simulink model "sim_tnse_2024_pos_ctrl"  (R2020a)
settings: Solver=ode4  StartTime=0.0  StopTime=30.0  FixedStep=0.01  RelTol=1e-3
values from neighbouring files (symbols this model uses):
  alfa_theta = 20    [init_tnse_2024_pos_ctrl.m]
  c1 = diag( [ 150.0, 120.0, 120.0 ] )    [init_tnse_2024_pos_ctrl.m]
  c1_diff_sigma_bar_v = diag([25; 30; 20])    [init_tnse_2024_pos_ctrl.m]
  c1v = diag([5.8; 6.5; 6.5])    [init_tnse_2024_pos_ctrl.m]
  c2 = diag( [ 80.0, 50.0, 50.0 ] )    [init_tnse_2024_pos_ctrl.m]
  c2_diff_sigma_bar_v = diag([50; 50; 10])    [init_tnse_2024_pos_ctrl.m]
  c2v = diag([5.8; 6.5; 6.5])    [init_tnse_2024_pos_ctrl.m]
  c3_diff_sigma_bar_v = diag([15; 15; 10])    [init_tnse_2024_pos_ctrl.m]
  c3v = diag([4.8; 6.4; 6.0])    [init_tnse_2024_pos_ctrl.m]
  dp_aa_t = 0.2 * ones(3, 5) + ( 1.0 - 0.2 ) * rand(3, 5)    [init_tnse_2024_pos_ctrl.m]
  dp_ff_t = [ 0.4 * ones(1, 5) + ( 1.0 - 0.4 ) * rand(1, 5);                      0.4 * ones(1, 5) + ( 1.0 - 0.4 ) * rand(1, 5);                      0.2 * ones(1, 5) + ( 0.6 - 0.2 ) * rand(1, 5) ]    [init_tnse_2024_pos_ctrl.m]
  dp_phi_t = ( - pi / 2 ) * ones(3, 5) + ( pi / 2 - ( - pi / 2 ) ) * rand(3, 5)    [init_tnse_2024_pos_ctrl.m]
  eps0 = [0.05; 0.01; 0.01]    [init_tnse_2024_pos_ctrl.m]
  etai_0 = zeros(3,5)    [init_tnse_2024_pos_ctrl.m]
  kai0 = [15; 10; 10]    [init_tnse_2024_pos_ctrl.m]
  kai_1_t = 0.02    [init_tnse_2024_pos_ctrl.m]
  kai_3_t = 0.1    [init_tnse_2024_pos_ctrl.m]
  ksii_0 = zeros(3,5)    [init_tnse_2024_pos_ctrl.m]
  lam0 = [15; 10; 10]    [init_tnse_2024_pos_ctrl.m]
  Lamd_diff_sigma_bar_v = 0.5    [init_tnse_2024_pos_ctrl.m]
  mass_i = zeros(1,NF)    [init_tnse_2024_pos_ctrl.m]
  Mii = diag([1;0;0;0;1])    [init_tnse_2024_pos_ctrl.m]
  pos0 = zeros(3, 1)    [init_tnse_2024_pos_ctrl.m]
  PZ0 = P0(3)    [init_tnse_2024_pos_ctrl.m]
  PZ1 = 10    [init_tnse_2024_pos_ctrl.m]
  Qci_init = repmat([1;0;0;0],1,NF)    [init_tnse_2024_pos_ctrl.m]
  R0 = 4    [init_tnse_2024_pos_ctrl.m]
  R1 = 8    [init_tnse_2024_pos_ctrl.m]
  Rx2 = 10    [init_tnse_2024_pos_ctrl.m]
  Ry2 = 6    [init_tnse_2024_pos_ctrl.m]
  Rz2 = 4    [init_tnse_2024_pos_ctrl.m]
  sat_sr_low = [-30, -30, -30]    [init_tnse_2024_pos_ctrl.m]
  sat_sr_up = [30, 30, 30]    [init_tnse_2024_pos_ctrl.m]
  T0 = 0    [init_tnse_2024_pos_ctrl.m]
  T1 = tseq1    (= 10)    [init_tnse_2024_pos_ctrl.m]
  T12 = tseq1 + tseq12    (= 20)    [init_tnse_2024_pos_ctrl.m]
  T2 = tseq1 + tseq12 + tseq2    (= 30)    [init_tnse_2024_pos_ctrl.m]
  theta0 = ( 2 / 5 ) * pi    (= 1.25663706144)    [init_tnse_2024_pos_ctrl.m]
  vel0 = zeros(3, 1)    [init_tnse_2024_pos_ctrl.m]
  Wij = [0,0,1,0,0;              0,0,1,1,0;              1,0,0,0,1;              0,1,1,0,0;              0,0,1,0,0]    [init_tnse_2024_pos_ctrl.m]
  X1 = 8    [init_tnse_2024_pos_ctrl.m]
  X2 = 2    [init_tnse_2024_pos_ctrl.m]
  X3 = 3    [init_tnse_2024_pos_ctrl.m]
  Y1 = 10    [init_tnse_2024_pos_ctrl.m]
  Y2 = 2    [init_tnse_2024_pos_ctrl.m]
  Y3 = 4    [init_tnse_2024_pos_ctrl.m]
  Z1 = 4    [init_tnse_2024_pos_ctrl.m]
  Z2 = -6    [init_tnse_2024_pos_ctrl.m]
  Z3 = 2    [init_tnse_2024_pos_ctrl.m]
  zeta_diff_sigma_bar_v = 0.08    [init_tnse_2024_pos_ctrl.m]
undefined symbols (not defined in the file or in its folder): cal_frac_squ, p_alfav1, p_alfav2, q_alfav1, q_alfav2
(part 3 of 4)

== matlab function sim_tnse_2024_pos_ctrl/cal differentiator d_sigma_bar_v_hat agent 4/cal sig ==
  data: x input; z output; y input
function z = fcn(x, y)
z = x(:) .* sign(y(:));

== matlab function sim_tnse_2024_pos_ctrl/Phi_sec_sigma_i agent 1 ==
  data: sigma_i_vec input; Phi_sec_sigma_1 output
function Phi_sec_sigma_1 = fcn(sigma_i_vec)
%%%% 跟随者期望速度分布式观测器
iiuav = 1;
Phi_sec_sigma_1 = diag( [ sech( sigma_i_vec(1,iiuav) ) ^ 2, ...
                                                sech( sigma_i_vec(2,iiuav) ) ^ 2, ...
                                                sech( sigma_i_vec(3,iiuav) ) ^ 2 ] );

== matlab function sim_tnse_2024_pos_ctrl/cal differentiator d_sigma_bar_v_hat agent 4/cal sig1 ==
  data: x input; z output; y input
function z = fcn(x, y)
z = x(:) .* sign(y(:));

== matlab function sim_tnse_2024_pos_ctrl/cal differentiator d_sigma_bar_v_hat agent 4/cal sig2 ==
  data: x input; z output; y input
function z = fcn(x, y)
z = x(:) .* sign(y(:));

== matlab function sim_tnse_2024_pos_ctrl/cal differentiator d_sigma_bar_v_hat agent 4/cal sig3 ==
  data: x input; z output; y input
function z = fcn(x, y)
z = x(:) .* sign(y(:));

== matlab function sim_tnse_2024_pos_ctrl/cal differentiator d_sigma_bar_v_hat agent 4/cal sig4 ==
  data: x input; z output; y input
function z = fcn(x, y)
z = x(:) .* sign(y(:));

== matlab function sim_tnse_2024_pos_ctrl/cal differentiator d_sigma_bar_v_hat agent 4/cal sig5 ==
  data: x input; z output; y input
function z = fcn(x, y)
z = x(:) .* sign(y(:));

== matlab function sim_tnse_2024_pos_ctrl/cal differentiator d_sigma_bar_v_hat agent 4/choose sigma_bar_v ==
  data: x input; y output
function y = fcn(x)
iiuav = 4;
y = x(:,iiuav);

== matlab function sim_tnse_2024_pos_ctrl/cal differentiator d_sigma_bar_v_hat agent 4/trans to column20 ==
  data: x input; y output
function y = fcn(x)
y = x(:);

== matlab function sim_tnse_2024_pos_ctrl/cal differentiator d_sigma_bar_v_hat agent 4/trans to column21 ==
  data: x input; y output
function y = fcn(x)
y = x(:);

== matlab function sim_tnse_2024_pos_ctrl/cal differentiator d_sigma_bar_v_hat agent 4/trans to column22 ==
  data: x input; y output
function y = fcn(x)
y = x(:);

== matlab function sim_tnse_2024_pos_ctrl/cal differentiator d_sigma_bar_v_hat agent 4/trans to column23 ==
  data: x input; y output
function y = fcn(x)
y = x(:);

== matlab function sim_tnse_2024_pos_ctrl/Phi_sec_sigma_i agent 2 ==
  data: sigma_i_vec input; Phi_sec_sigma_2 output
function Phi_sec_sigma_2 = fcn(sigma_i_vec)
%%%% 跟随者期望速度分布式观测器
iiuav = 2;
Phi_sec_sigma_2 = diag( [ sech( sigma_i_vec(1,iiuav) ) ^ 2, ...
                                                sech( sigma_i_vec(2,iiuav) ) ^ 2, ...
                                                sech( sigma_i_vec(3,iiuav) ) ^ 2 ] );

== matlab function sim_tnse_2024_pos_ctrl/cal Rci from ui ==
  data: Rci output; mi_vec input; ui_vec input
function Rci = fcn(mi_vec, ui_vec)
Rci = zeros(3,3,5);
for iiuav = 1:5
    Rci(:,:,iiuav) = cal_Rc_with_u(mi_vec(iiuav), ui_vec(:,iiuav));
end

end

== matlab function sim_tnse_2024_pos_ctrl/cal differentiator d_sigma_bar_v_hat agent 4/trans to column24 ==
  data: x input; y output
function y = fcn(x)
y = x(:);

== matlab function sim_tnse_2024_pos_ctrl/cal differentiator d_sigma_bar_v_hat agent 4/trans to column25 ==
  data: x input; y output
function y = fcn(x)
y = x(:);

== matlab function sim_tnse_2024_pos_ctrl/cal differentiator d_sigma_bar_v_hat agent 5/cal differentiator ==
  data: c1 input; d_sigma_bar_v_hat output; d_dsigma_bar_v_hat output; d_d2sigma_bar_v_hat output; c2 input; c3 input; chi_t input; sigma_bar_v_sig_1 input; sigma_bar_v_sig_2 input; sigma_bar_v_sig_3 input; sigma_bar_v_sig_4 input; sigma_bar_v_sig_5 input; sigma_bar_v_sig_6 input; d_sigma_bar_v_hat input; d2_sigma_bar_v_hat input
function [d_sigma_bar_v_hat, d_dsigma_bar_v_hat, d_d2sigma_bar_v_hat] = fcn(c1, c2, c3, chi_t, sigma_bar_v_sig_1, sigma_bar_v_sig_2, sigma_bar_v_sig_3, ...
                                                                                                                                                sigma_bar_v_sig_4, sigma_bar_v_sig_5, sigma_bar_v_sig_6, d_sigma_bar_v_hat, d2_sigma_bar_v_hat)
d_d2sigma_bar_v_hat = -chi_t .* c1 * sigma_bar_v_sig_1(:) - (1 - chi_t) .* c1 * sigma_bar_v_sig_2(:);
d_dsigma_bar_v_hat = -chi_t .* c2 * sigma_bar_v_sig_3(:) - (1 - chi_t) .* c2 * sigma_bar_v_sig_4(:) + d2_sigma_bar_v_hat(:);
d_sigma_bar_v_hat = -chi_t .* c3 * sigma_bar_v_sig_5(:) - (1 - chi_t) .* c3 * sigma_bar_v_sig_6(:) + d_sigma_bar_v_hat(:);

== matlab function sim_tnse_2024_pos_ctrl/cal differentiator d_sigma_bar_v_hat agent 5/cal sig ==
  data: x input; z output; y input
function z = fcn(x, y)
z = x(:) .* sign(y(:));

== matlab function sim_tnse_2024_pos_ctrl/cal differentiator d_sigma_bar_v_hat agent 5/cal sig1 ==
  data: x input; z output; y input
function z = fcn(x, y)
z = x(:) .* sign(y(:));

== matlab function sim_tnse_2024_pos_ctrl/cal differentiator d_sigma_bar_v_hat agent 5/cal sig2 ==
  data: x input; z output; y input
function z = fcn(x, y)
z = x(:) .* sign(y(:));

== matlab function sim_tnse_2024_pos_ctrl/Phi_sec_sigma_i agent 3 ==
  data: sigma_i_vec input; Phi_sec_sigma_3 output
function Phi_sec_sigma_3 = fcn(sigma_i_vec)
%%%% 跟随者期望速度分布式观测器
iiuav = 3;
Phi_sec_sigma_3 = diag( [ sech( sigma_i_vec(1,iiuav) ) ^ 2, ...
                                                sech( sigma_i_vec(2,iiuav) ) ^ 2, ...
                                                sech( sigma_i_vec(3,iiuav) ) ^ 2 ] );

== matlab function sim_tnse_2024_pos_ctrl/cal differentiator d_sigma_bar_v_hat agent 5/cal sig3 ==
  data: x input; z output; y input
function z = fcn(x, y)
z = x(:) .* sign(y(:));

== matlab function sim_tnse_2024_pos_ctrl/cal differentiator d_sigma_bar_v_hat agent 5/cal sig4 ==
  data: x input; z output; y input
function z = fcn(x, y)
z = x(:) .* sign(y(:));

== matlab function sim_tnse_2024_pos_ctrl/cal differentiator d_sigma_bar_v_hat agent 5/cal sig5 ==
  data: x input; z output; y input
function z = fcn(x, y)
z = x(:) .* sign(y(:));

== matlab function sim_tnse_2024_pos_ctrl/cal differentiator d_sigma_bar_v_hat agent 5/choose sigma_bar_v ==
  data: x input; y output
function y = fcn(x)
iiuav = 5;
y = x(:,iiuav);

== matlab function sim_tnse_2024_pos_ctrl/cal differentiator d_sigma_bar_v_hat agent 5/trans to column20 ==
  data: x input; y output
function y = fcn(x)
y = x(:);

== matlab function sim_tnse_2024_pos_ctrl/cal differentiator d_sigma_bar_v_hat agent 5/trans to column21 ==
  data: x input; y output
function y = fcn(x)
y = x(:);

== matlab function sim_tnse_2024_pos_ctrl/cal differentiator d_sigma_bar_v_hat agent 5/trans to column22 ==
  data: x input; y output
function y = fcn(x)
y = x(:);

== matlab function sim_tnse_2024_pos_ctrl/cal differentiator d_sigma_bar_v_hat agent 5/trans to column23 ==
  data: x input; y output
function y = fcn(x)
y = x(:);

== matlab function sim_tnse_2024_pos_ctrl/cal differentiator d_sigma_bar_v_hat agent 5/trans to column24 ==
  data: x input; y output
function y = fcn(x)
y = x(:);

== matlab function sim_tnse_2024_pos_ctrl/cal differentiator d_sigma_bar_v_hat agent 5/trans to column25 ==
  data: x input; y output
function y = fcn(x)
y = x(:);

== matlab function sim_tnse_2024_pos_ctrl/Phi_sec_sigma_i agent 4 ==
  data: sigma_i_vec input; Phi_sec_sigma_4 output
function Phi_sec_sigma_4 = fcn(sigma_i_vec)
%%%% 跟随者期望速度分布式观测器
iiuav = 4;
Phi_sec_sigma_4 = diag( [ sech( sigma_i_vec(1,iiuav) ) ^ 2, ...
                                                sech( sigma_i_vec(2,iiuav) ) ^ 2, ...
                                                sech( sigma_i_vec(3,iiuav) ) ^ 2 ] );

== matlab function sim_tnse_2024_pos_ctrl/combine d_sigma_bar_v_est ==
  data: d_sigma_bar_v_est_1 input; d_sigma_bar_v_est_2 input; d_sigma_bar_v_est_3 input; d_sigma_bar_v_est_4 input; d_sigma_bar_v_est_5 input; d_sigma_bar_v_vec output
function d_sigma_bar_v_vec  = fcn(d_sigma_bar_v_est_1, d_sigma_bar_v_est_2, d_sigma_bar_v_est_3, d_sigma_bar_v_est_4, d_sigma_bar_v_est_5)
%%%% 合并用微分器求得的虚拟速度控制量导数
d_sigma_bar_v_vec = [d_sigma_bar_v_est_1(:), d_sigma_bar_v_est_2(:), d_sigma_bar_v_est_3(:), d_sigma_bar_v_est_4(:), d_sigma_bar_v_est_5(:)];

== matlab function sim_tnse_2024_pos_ctrl/cal abs 21 ==
  data: x input; y output
function y = fcn(x)
y = abs(x(:));

== matlab function sim_tnse_2024_pos_ctrl/cal abs 22 ==
  data: x input; y output
function y = fcn(x)
y = abs(x(:));

== matlab function sim_tnse_2024_pos_ctrl/choose ksi_est_err 21 ==
  data: x input; y output
function y = fcn(x)
iiuav = 1;
y = x(:,iiuav);

== matlab function sim_tnse_2024_pos_ctrl/choose ksi_est_err 22 ==
  data: x input; y output
function y = fcn(x)
iiuav = 1;
y = x(:,iiuav);

== matlab function sim_tnse_2024_pos_ctrl/trans to column20 ==
  data: x input; y output
function y = fcn(x)
y = x(:);

== matlab function sim_tnse_2024_pos_ctrl/trans to column21 ==
  data: x input; y output
function y = fcn(x)
y = x(:);

== matlab function sim_tnse_2024_pos_ctrl/cal theta_sigma_bar_v_tilt agent 1 ==
  data: alfa_theta input; sigma_bar_v_tilt_squ_1_1 input; theta_sigma_bar_v_tilt_1_1 output; sigma_bar_v_tilt_squ_2_1 input; sigma_bar_v_tilt_vec input; theta_sigma_bar_v_tilt_2_1 output
function [theta_sigma_bar_v_tilt_1_1, theta_sigma_bar_v_tilt_2_1] = fcn(alfa_theta, sigma_bar_v_tilt_squ_1_1, sigma_bar_v_tilt_squ_2_1, sigma_bar_v_tilt_vec)
%%%% 计算平滑递增函数
iiuav = 1;
theta_sigma_bar_v_tilt_1_1 = sigma_bar_v_tilt_squ_1_1(:) .* ( -1 + 2 ./ ( 1 + exp( -alfa_theta .* sigma_bar_v_tilt_vec(:,iiuav) ) ) );
theta_sigma_bar_v_tilt_2_1 = sigma_bar_v_tilt_squ_2_1(:) .* ( -1 + 2 ./ ( 1 + exp( -alfa_theta .* sigma_bar_v_tilt_vec(:,iiuav) ) ) );

== matlab function sim_tnse_2024_pos_ctrl/cal abs 23 ==
  data: x input; y output
function y = fcn(x)
y = abs(x(:));

== matlab function sim_tnse_2024_pos_ctrl/Phi_sec_sigma_i agent 5 ==
  data: sigma_i_vec input; Phi_sec_sigma_5 output
function Phi_sec_sigma_5 = fcn(sigma_i_vec)
%%%% 跟随者期望速度分布式观测器
iiuav = 5;
Phi_sec_sigma_5 = diag( [ sech( sigma_i_vec(1,iiuav) ) ^ 2, ...
                                                sech( sigma_i_vec(2,iiuav) ) ^ 2, ...
                                                sech( sigma_i_vec(3,iiuav) ) ^ 2 ] );

== matlab function sim_tnse_2024_pos_ctrl/cal abs 24 ==
  data: x input; y output
function y = fcn(x)
y = abs(x(:));

== matlab function sim_tnse_2024_pos_ctrl/cal theta_sigma_bar_v_tilt agent 2 ==
  data: alfa_theta input; sigma_bar_v_tilt_squ_1_2 input; theta_sigma_bar_v_tilt_1_2 output; sigma_bar_v_tilt_squ_2_2 input; sigma_bar_v_tilt_vec input; theta_sigma_bar_v_tilt_2_2 output
function [theta_sigma_bar_v_tilt_1_2, theta_sigma_bar_v_tilt_2_2] = fcn(alfa_theta, sigma_bar_v_tilt_squ_1_2, sigma_bar_v_tilt_squ_2_2, sigma_bar_v_tilt_vec)
%%%% 计算平滑递增函数
iiuav = 2;
theta_sigma_bar_v_tilt_1_2 = sigma_bar_v_tilt_squ_1_2(:) .* ( -1 + 2 ./ ( 1 + exp( -alfa_theta .* sigma_bar_v_tilt_vec(:,iiuav) ) ) );
theta_sigma_bar_v_tilt_2_2 = sigma_bar_v_tilt_squ_2_2(:) .* ( -1 + 2 ./ ( 1 + exp( -alfa_theta .* sigma_bar_v_tilt_vec(:,iiuav) ) ) );

== matlab function sim_tnse_2024_pos_ctrl/choose ksi_est_err 23 ==
  data: x input; y output
function y = fcn(x)
iiuav = 2;
y = x(:,iiuav);

== matlab function sim_tnse_2024_pos_ctrl/choose ksi_est_err 24 ==
  data: x input; y output
function y = fcn(x)
iiuav = 2;
y = x(:,iiuav);

== matlab function sim_tnse_2024_pos_ctrl/trans to column22 ==
  data: x input; y output
function y = fcn(x)
y = x(:);

== matlab function sim_tnse_2024_pos_ctrl/trans to column23 ==
  data: x input; y output
function y = fcn(x)
y = x(:);

== matlab function sim_tnse_2024_pos_ctrl/cal abs 25 ==
  data: x input; y output
function y = fcn(x)
y = abs(x(:));

== matlab function sim_tnse_2024_pos_ctrl/cal abs 26 ==
  data: x input; y output
function y = fcn(x)
y = abs(x(:));

== matlab function sim_tnse_2024_pos_ctrl/cal theta_sigma_bar_v_tilt agent 3 ==
  data: alfa_theta input; sigma_bar_v_tilt_squ_1_3 input; theta_sigma_bar_v_tilt_1_3 output; sigma_bar_v_tilt_squ_2_3 input; sigma_bar_v_tilt_vec input; theta_sigma_bar_v_tilt_2_3 output
function [theta_sigma_bar_v_tilt_1_3, theta_sigma_bar_v_tilt_2_3] = fcn(alfa_theta, sigma_bar_v_tilt_squ_1_3, sigma_bar_v_tilt_squ_2_3, sigma_bar_v_tilt_vec)
%%%% 计算平滑递增函数
iiuav = 3;
theta_sigma_bar_v_tilt_1_3 = sigma_bar_v_tilt_squ_1_3(:) .* ( -1 + 2 ./ ( 1 + exp( -alfa_theta .* sigma_bar_v_tilt_vec(:,iiuav) ) ) );
theta_sigma_bar_v_tilt_2_3 = sigma_bar_v_tilt_squ_2_3(:) .* ( -1 + 2 ./ ( 1 + exp( -alfa_theta .* sigma_bar_v_tilt_vec(:,iiuav) ) ) );

== matlab function sim_tnse_2024_pos_ctrl/combine betai ==
  data: beta_hat_1 input; beta_hat_vec output; beta_hat_2 input; beta_hat_3 input; beta_hat_4 input; beta_hat_5 input
function beta_hat_vec  = fcn(beta_hat_1, beta_hat_2, beta_hat_3, beta_hat_4, beta_hat_5)
%%%% 合并自适应律
beta_hat_vec = [beta_hat_1, beta_hat_2, beta_hat_3, beta_hat_4, beta_hat_5];

== matlab function sim_tnse_2024_pos_ctrl/choose ksi_est_err 25 ==
  data: x input; y output
function y = fcn(x)
iiuav = 3;
y = x(:,iiuav);

== matlab function sim_tnse_2024_pos_ctrl/choose ksi_est_err 26 ==
  data: x input; y output
function y = fcn(x)
iiuav = 3;
y = x(:,iiuav);

== matlab function sim_tnse_2024_pos_ctrl/trans to column24 ==
  data: x input; y output
function y = fcn(x)
y = x(:);

== matlab function sim_tnse_2024_pos_ctrl/trans to column25 ==
  data: x input; y output
function y = fcn(x)
y = x(:);

== matlab function sim_tnse_2024_pos_ctrl/cal abs 27 ==
  data: x input; y output
function y = fcn(x)
y = abs(x(:));

== matlab function sim_tnse_2024_pos_ctrl/cal abs 28 ==
  data: x input; y output
function y = fcn(x)
y = abs(x(:));

== matlab function sim_tnse_2024_pos_ctrl/cal theta_sigma_bar_v_tilt agent 4 ==
  data: alfa_theta input; sigma_bar_v_tilt_squ_1_4 input; theta_sigma_bar_v_tilt_1_4 output; sigma_bar_v_tilt_squ_2_4 input; sigma_bar_v_tilt_vec input; theta_sigma_bar_v_tilt_2_4 output
function [theta_sigma_bar_v_tilt_1_4, theta_sigma_bar_v_tilt_2_4] = fcn(alfa_theta, sigma_bar_v_tilt_squ_1_4, sigma_bar_v_tilt_squ_2_4, sigma_bar_v_tilt_vec)
%%%% 计算平滑递增函数
iiuav = 4;
theta_sigma_bar_v_tilt_1_4 = sigma_bar_v_tilt_squ_1_4(:) .* ( -1 + 2 ./ ( 1 + exp( -alfa_theta .* sigma_bar_v_tilt_vec(:,iiuav) ) ) );
theta_sigma_bar_v_tilt_2_4 = sigma_bar_v_tilt_squ_2_4(:) .* ( -1 + 2 ./ ( 1 + exp( -alfa_theta .* sigma_bar_v_tilt_vec(:,iiuav) ) ) );

== matlab function sim_tnse_2024_pos_ctrl/choose ksi_est_err 27 ==
  data: x input; y output
function y = fcn(x)
iiuav = 4;
y = x(:,iiuav);

== matlab function sim_tnse_2024_pos_ctrl/choose ksi_est_err 28 ==
  data: x input; y output
function y = fcn(x)
iiuav = 4;
y = x(:,iiuav);

== matlab function sim_tnse_2024_pos_ctrl/trans to column26 ==
  data: x input; y output
function y = fcn(x)
y = x(:);

== matlab function sim_tnse_2024_pos_ctrl/trans to column27 ==
  data: x input; y output
function y = fcn(x)
y = x(:);

== matlab function sim_tnse_2024_pos_ctrl/cal abs 29 ==
  data: x input; y output
function y = fcn(x)
y = abs(x(:));

== matlab function sim_tnse_2024_pos_ctrl/cal abs 30 ==
  data: x input; y output
function y = fcn(x)
y = abs(x(:));

== matlab function sim_tnse_2024_pos_ctrl/cal theta_sigma_bar_v_tilt agent 5 ==
  data: alfa_theta input; sigma_bar_v_tilt_squ_1_5 input; theta_sigma_bar_v_tilt_1_5 output; sigma_bar_v_tilt_squ_2_5 input; sigma_bar_v_tilt_vec input; theta_sigma_bar_v_tilt_2_5 output
function [theta_sigma_bar_v_tilt_1_5, theta_sigma_bar_v_tilt_2_5] = fcn(alfa_theta, sigma_bar_v_tilt_squ_1_5, sigma_bar_v_tilt_squ_2_5, sigma_bar_v_tilt_vec)
%%%% 计算平滑递增函数
iiuav = 5;
theta_sigma_bar_v_tilt_1_5 = sigma_bar_v_tilt_squ_1_5(:) .* ( -1 + 2 ./ ( 1 + exp( -alfa_theta .* sigma_bar_v_tilt_vec(:,iiuav) ) ) );
theta_sigma_bar_v_tilt_2_5 = sigma_bar_v_tilt_squ_2_5(:) .* ( -1 + 2 ./ ( 1 + exp( -alfa_theta .* sigma_bar_v_tilt_vec(:,iiuav) ) ) );

== matlab function sim_tnse_2024_pos_ctrl/update betai agent 1 ==
  data: eps0 input; d_beta_hat_1 output; Wij input; Mii input; tsim input; u0 input; rho_hat_vec input
function d_beta_hat_1 = fcn(eps0, Wij, Mii, tsim, u0, rho_hat_vec)
%%%% 自适应律
iiuav = 1;
err_rho = Mii(iiuav, iiuav) * ( rho_hat_vec(:,iiuav) - u0(:) );
for jjuav = 1:5
    err_rho = err_rho + Wij(iiuav, jjuav) * ( rho_hat_vec(:,iiuav) - rho_hat_vec(:,jjuav) );
end
d_beta_hat_1 = ( err_rho(:)' ) * tanh( err_rho(:) ./ exp( -eps0 * tsim ) );

== matlab function sim_tnse_2024_pos_ctrl/choose ksi_est_err 29 ==
  data: x input; y output
function y = fcn(x)
iiuav = 5;
y = x(:,iiuav);

== matlab function sim_tnse_2024_pos_ctrl/choose ksi_est_err 30 ==
  data: x input; y output
function y = fcn(x)
iiuav = 5;
y = x(:,iiuav);

== matlab function sim_tnse_2024_pos_ctrl/trans to column28 ==
  data: x input; y output
function y = fcn(x)
y = x(:);

== matlab function sim_tnse_2024_pos_ctrl/trans to column29 ==
  data: x input; y output
function y = fcn(x)
y = x(:);

== matlab function sim_tnse_2024_pos_ctrl/combine theta_sigma_bar_v_tilt ==
  data: theta_sigma_bar_v_tilt_1_1 input; theta_sigma_bar_v_tilt_1_2 input; theta_sigma_bar_v_tilt_1_3 input; theta_sigma_bar_v_tilt_1_4 input; theta_sigma_bar_v_tilt_1_5 input; theta_sigma_bar_v_tilt_1_vec output; theta_sigma_bar_v_tilt_2_1 input; theta_sigma_bar_v_tilt_2_vec output; theta_sigma_bar_v_tilt_2_2 input; theta_sigma_bar_v_tilt_2_3 input; theta_sigma_bar_v_tilt_2_4 input; theta_sigma_bar_v_tilt_2_5 input
function [theta_sigma_bar_v_tilt_1_vec, theta_sigma_bar_v_tilt_2_vec]  = fcn(theta_sigma_bar_v_tilt_1_1, theta_sigma_bar_v_tilt_1_2, theta_sigma_bar_v_tilt_1_3, theta_sigma_bar_v_tilt_1_4, theta_sigma_bar_v_tilt_1_5, ...
                                                                                                                                            theta_sigma_bar_v_tilt_2_1, theta_sigma_bar_v_tilt_2_2, theta_sigma_bar_v_tilt_2_3, theta_sigma_bar_v_tilt_2_4, theta_sigma_bar_v_tilt_2_5)
%%%% 合并领导者位置观测器输出结果
theta_sigma_bar_v_tilt_1_vec = [theta_sigma_bar_v_tilt_1_1(:), theta_sigma_bar_v_tilt_1_2(:), theta_sigma_bar_v_tilt_1_3(:), theta_sigma_bar_v_tilt_1_4(:), theta_sigma_bar_v_tilt_1_5(:)];
theta_sigma_bar_v_tilt_2_vec = [theta_sigma_bar_v_tilt_2_1(:), theta_sigma_bar_v_tilt_2_2(:), theta_sigma_bar_v_tilt_2_3(:), theta_sigma_bar_v_tilt_2_4(:), theta_sigma_bar_v_tilt_2_5(:)];

== matlab function sim_tnse_2024_pos_ctrl/cal sigma_bar_v_hat agent 1 ==
  data: c1v input; c2v input; theta_sigma_bar_v_tilt_1_vec input; d_sigma_bar_v_hat_1 output; theta_sigma_bar_v_tilt_2_vec input; d_sigma_bar_v_vec input
function d_sigma_bar_v_hat_1 = fcn(c1v, c2v, theta_sigma_bar_v_tilt_1_vec, theta_sigma_bar_v_tilt_2_vec, d_sigma_bar_v_vec)
%%%% 计算扰动观测器中虚拟速度控制量观测值sigma_v_hat的微分方程
iiuav = 1;
d_sigma_bar_v_hat_1 = d_sigma_bar_v_vec(:,iiuav) + ...
                                            c1v * theta_sigma_bar_v_tilt_1_vec(:,iiuav) + ...
                                            c2v * theta_sigma_bar_v_tilt_2_vec(:,iiuav);

== matlab function sim_tnse_2024_pos_ctrl/cal sigma_bar_v_hat agent 2 ==
  data: c1v input; c2v input; theta_sigma_bar_v_tilt_1_vec input; d_sigma_bar_v_hat_2 output; theta_sigma_bar_v_tilt_2_vec input; d_sigma_bar_v_vec input
function d_sigma_bar_v_hat_2 = fcn(c1v, c2v, theta_sigma_bar_v_tilt_1_vec, theta_sigma_bar_v_tilt_2_vec, d_sigma_bar_v_vec)
%%%% 计算扰动观测器中虚拟速度控制量观测值sigma_v_hat的微分方程
iiuav = 2;
d_sigma_bar_v_hat_2 = d_sigma_bar_v_vec(:,iiuav) + ...
                                            c1v * theta_sigma_bar_v_tilt_1_vec(:,iiuav) + ...
                                            c2v * theta_sigma_bar_v_tilt_2_vec(:,iiuav);

== matlab function sim_tnse_2024_pos_ctrl/cal sigma_bar_v_hat agent 3 ==
  data: c1v input; c2v input; theta_sigma_bar_v_tilt_1_vec input; d_sigma_bar_v_hat_3 output; theta_sigma_bar_v_tilt_2_vec input; d_sigma_bar_v_vec input
function d_sigma_bar_v_hat_3 = fcn(c1v, c2v, theta_sigma_bar_v_tilt_1_vec, theta_sigma_bar_v_tilt_2_vec, d_sigma_bar_v_vec)
%%%% 计算扰动观测器中虚拟速度控制量观测值sigma_v_hat的微分方程
iiuav = 3;
d_sigma_bar_v_hat_3 = d_sigma_bar_v_vec(:,iiuav) + ...
                                            c1v * theta_sigma_bar_v_tilt_1_vec(:,iiuav) + ...
                                            c2v * theta_sigma_bar_v_tilt_2_vec(:,iiuav);

== matlab function sim_tnse_2024_pos_ctrl/cal sigma_bar_v_hat agent 4 ==
  data: c1v input; c2v input; theta_sigma_bar_v_tilt_1_vec input; d_sigma_bar_v_hat_4 output; theta_sigma_bar_v_tilt_2_vec input; d_sigma_bar_v_vec input
function d_sigma_bar_v_hat_4 = fcn(c1v, c2v, theta_sigma_bar_v_tilt_1_vec, theta_sigma_bar_v_tilt_2_vec, d_sigma_bar_v_vec)
%%%% 计算扰动观测器中虚拟速度控制量观测值sigma_v_hat的微分方程
iiuav = 4;
d_sigma_bar_v_hat_4 = d_sigma_bar_v_vec(:,iiuav) + ...
                                            c1v * theta_sigma_bar_v_tilt_1_vec(:,iiuav) + ...
                                            c2v * theta_sigma_bar_v_tilt_2_vec(:,iiuav);

== matlab function sim_tnse_2024_pos_ctrl/cal sigma_bar_v_hat agent 5 ==
  data: c1v input; c2v input; theta_sigma_bar_v_tilt_1_vec input; d_sigma_bar_v_hat_5 output; theta_sigma_bar_v_tilt_2_vec input; d_sigma_bar_v_vec input
function d_sigma_bar_v_hat_5 = fcn(c1v, c2v, theta_sigma_bar_v_tilt_1_vec, theta_sigma_bar_v_tilt_2_vec, d_sigma_bar_v_vec)
%%%% 计算扰动观测器中虚拟速度控制量观测值sigma_v_hat的微分方程
iiuav = 5;
d_sigma_bar_v_hat_5 = d_sigma_bar_v_vec(:,iiuav) + ...
                                            c1v * theta_sigma_bar_v_tilt_1_vec(:,iiuav) + ...
                                            c2v * theta_sigma_bar_v_tilt_2_vec(:,iiuav);

== matlab function sim_tnse_2024_pos_ctrl/cal combine sigma_bar_v_tilt ==
  data: sigma_bar_v_vec input; sigma_bar_v_hat_vec input; sigma_bar_v_tilt_vec output
function sigma_bar_v_tilt_vec = fcn(sigma_bar_v_vec, sigma_bar_v_hat_vec)
%%%% 计算虚拟速度观测误差sigma_bar_v_tilt
sigma_bar_v_tilt_vec = zeros(3,5);
for iiuav = 1:5
    sigma_bar_v_tilt_vec(:,iiuav) = sigma_bar_v_vec(:,iiuav) - sigma_bar_v_hat_vec(:,iiuav);
end

== matlab function sim_tnse_2024_pos_ctrl/combine sigma_bar_v_hat ==
  data: sigma_bar_v_hat_1 input; sigma_bar_v_hat_2 input; sigma_bar_v_hat_3 input; sigma_bar_v_hat_4 input; sigma_bar_v_hat_5 input; sigma_bar_v_hat_vec output
function sigma_bar_v_hat_vec  = fcn(sigma_bar_v_hat_1, sigma_bar_v_hat_2, sigma_bar_v_hat_3, sigma_bar_v_hat_4, sigma_bar_v_hat_5)
%%%% 合并虚拟速度控制量观测值sigma_bar_v_hat
sigma_bar_v_hat_vec = [sigma_bar_v_hat_1(:), sigma_bar_v_hat_2(:), sigma_bar_v_hat_3(:), sigma_bar_v_hat_4(:), sigma_bar_v_hat_5(:)];

== matlab function sim_tnse_2024_pos_ctrl/update betai agent 2 ==
  data: eps0 input; d_beta_hat_2 output; Wij input; Mii input; tsim input; u0 input; rho_hat_vec input
function d_beta_hat_2 = fcn(eps0, Wij, Mii, tsim, u0, rho_hat_vec)
%%%% 自适应律
iiuav = 2;
err_rho = Mii(iiuav, iiuav) * ( rho_hat_vec(:,iiuav) - u0(:) );
for jjuav = 1:5
    err_rho = err_rho + Wij(iiuav, jjuav) * ( rho_hat_vec(:,iiuav) - rho_hat_vec(:,jjuav) );
end
d_beta_hat_2 = ( err_rho(:)' ) * tanh( err_rho(:) ./ exp( -eps0 * tsim ) );

== matlab function sim_tnse_2024_pos_ctrl/cal dp_hat agent 1 ==
  data: c3v input; d_sigma_bar_v_vec input; sigma_bar_v_hat_vec input; dp_hat_1 output
function dp_hat_1 = fcn(c3v, d_sigma_bar_v_vec, sigma_bar_v_hat_vec)
%%%% 计算扰动观测值dp_hat
iiuav = 1;
dp_hat_1 = d_sigma_bar_v_vec(:,iiuav) + c3v * sigma_bar_v_hat_vec(:,iiuav);

== matlab function sim_tnse_2024_pos_ctrl/cal dp_hat agent 2 ==
  data: c3v input; d_sigma_bar_v_vec input; sigma_bar_v_hat_vec input; dp_hat_2 output
function dp_hat_2 = fcn(c3v, d_sigma_bar_v_vec, sigma_bar_v_hat_vec)
%%%% 计算扰动观测值dp_hat
iiuav = 2;
dp_hat_2 = d_sigma_bar_v_vec(:,iiuav) + c3v * sigma_bar_v_hat_vec(:,iiuav);

== matlab function sim_tnse_2024_pos_ctrl/cal dp_hat agent 3 ==
  data: c3v input; d_sigma_bar_v_vec input; sigma_bar_v_hat_vec input; dp_hat_3 output
function dp_hat_3 = fcn(c3v, d_sigma_bar_v_vec, sigma_bar_v_hat_vec)
%%%% 计算扰动观测值dp_hat
iiuav = 3;
dp_hat_3 = d_sigma_bar_v_vec(:,iiuav) + c3v * sigma_bar_v_hat_vec(:,iiuav);

== matlab function sim_tnse_2024_pos_ctrl/cal dp_hat agent 4 ==
  data: c3v input; d_sigma_bar_v_vec input; sigma_bar_v_hat_vec input; dp_hat_4 output
function dp_hat_4 = fcn(c3v, d_sigma_bar_v_vec, sigma_bar_v_hat_vec)
%%%% 计算扰动观测值dp_hat
iiuav = 4;
dp_hat_4 = d_sigma_bar_v_vec(:,iiuav) + c3v * sigma_bar_v_hat_vec(:,iiuav);

== matlab function sim_tnse_2024_pos_ctrl/cal dp_hat agent 5 ==
  data: c3v input; d_sigma_bar_v_vec input; sigma_bar_v_hat_vec input; dp_hat_5 output
function dp_hat_5 = fcn(c3v, d_sigma_bar_v_vec, sigma_bar_v_hat_vec)
%%%% 计算扰动观测值dp_hat
iiuav = 5;
dp_hat_5 = d_sigma_bar_v_vec(:,iiuav) + c3v * sigma_bar_v_hat_vec(:,iiuav);

== matlab function sim_tnse_2024_pos_ctrl/combine dp_hat ==
  data: dp_hat_1 input; dp_hat_2 input; dp_hat_3 input; dp_hat_4 input; dp_hat_5 input; dp_hat_vec output
function dp_hat_vec  = fcn(dp_hat_1, dp_hat_2, dp_hat_3, dp_hat_4, dp_hat_5)
%%%% 合并扰动观测值dp_hat
dp_hat_vec = [dp_hat_1(:), dp_hat_2(:), dp_hat_3(:), dp_hat_4(:), dp_hat_5(:)];

== matlab function sim_tnse_2024_pos_ctrl/cal ui agent 1 ==
  data: c1 input; c2 input; sat_sr_up input; sat_sr_low input; ui_1 output; rho_hat_vec input; dp_hat_vec input; si_vec input; ri_vec input
function ui_1 = fcn(c1, c2, sat_sr_up, sat_sr_low, rho_hat_vec, dp_hat_vec, si_vec, ri_vec)
%%%% 计算控制输入ui
iiuav = 1;
g0 = 9.80663;
e3 = [0;0;1];
sat_si_ri = zeros(3,1);
sat_ri = zeros(3,1);
c_mul_si_ri = c1 * ( si_vec(:,iiuav) + ri_vec(:,iiuav) );
c_mul_ri = c2 * ri_vec(:,iiuav);
for jj = 1:3
    if c_mul_si_ri(jj) < sat_sr_low(jj)
        sat_si_ri(jj) = sat_sr_low(jj);
    elseif c_mul_si_ri(jj) > sat_sr_up(jj)
        sat_si_ri(jj) = sat_sr_up(jj);
    else
        sat_si_ri(jj) = c_mul_ri(jj);
    end
    if c_mul_ri(jj) < sat_sr_low(jj)
        sat_ri(jj) = sat_sr_low(jj);
    elseif c_mul_ri(jj) > sat_sr_up(jj)
        sat_ri(jj) = sat_sr_up(jj);
    else
        sat_ri(jj) = c_mul_ri(jj);
    end
end
ui_1 = g0 * e3 + rho_hat_vec(:,iiuav) - dp_hat_vec(:,iiuav) ...
            - sat_si_ri(:) - sat_ri(:);

== matlab function sim_tnse_2024_pos_ctrl/combine ui ==
  data: ui_1 input; ui_2 input; ui_3 input; ui_4 input; ui_5 input; ui_vec output
function ui_vec  = fcn(ui_1, ui_2, ui_3, ui_4, ui_5)
%%%% 合并控制输入ui
ui_vec = [ui_1(:), ui_2(:), ui_3(:), ui_4(:), ui_5(:)];

== matlab function sim_tnse_2024_pos_ctrl/cal disturbance observation error dp_tilt ==
  data: dp_vec input; dp_tilt_vec output; dp_hat_vec input
function dp_tilt_vec = fcn(dp_vec, dp_hat_vec)
%%%% 计算扰动观测器估计误差dp_tilt
dp_tilt_vec = zeros(3,5);
for iiuav = 1:5
    dp_tilt_vec(:,iiuav) = dp_vec(:,iiuav) - dp_hat_vec(:,iiuav);
end

== matlab function sim_tnse_2024_pos_ctrl/combine Phi_sec_sigma_i ==
  data: Phi_sec_sigma_1 input; Phi_sec_sigma_vec output; Phi_sec_sigma_2 input; Phi_sec_sigma_3 input; Phi_sec_sigma_4 input; Phi_sec_sigma_5 input
function Phi_sec_sigma_vec  = fcn(Phi_sec_sigma_1, Phi_sec_sigma_2, Phi_sec_sigma_3, Phi_sec_sigma_4, Phi_sec_sigma_5)
%%%% 合并领导者位置观测器输出结果
Phi_sec_sigma_vec = zeros(3,3,5);
Phi_sec_sigma_vec(:,:,1) = Phi_sec_sigma_1;
Phi_sec_sigma_vec(:,:,2) = Phi_sec_sigma_2;
Phi_sec_sigma_vec(:,:,3) = Phi_sec_sigma_3;
Phi_sec_sigma_vec(:,:,4) = Phi_sec_sigma_4;
Phi_sec_sigma_vec(:,:,5) = Phi_sec_sigma_5;

== matlab function sim_tnse_2024_pos_ctrl/update betai agent 3 ==
  data: eps0 input; d_beta_hat_3 output; Wij input; Mii input; tsim input; u0 input; rho_hat_vec input
function d_beta_hat_3 = fcn(eps0, Wij, Mii, tsim, u0, rho_hat_vec)
%%%% 自适应律
iiuav = 3;
err_rho = Mii(iiuav, iiuav) * ( rho_hat_vec(:,iiuav) - u0(:) );
for jjuav = 1:5
    err_rho = err_rho + Wij(iiuav, jjuav) * ( rho_hat_vec(:,iiuav) - rho_hat_vec(:,jjuav) );
end
d_beta_hat_3 = ( err_rho(:)' ) * tanh( err_rho(:) ./ exp( -eps0 * tsim ) );

== matlab function sim_tnse_2024_pos_ctrl/update betai agent 4 ==
  data: eps0 input; d_beta_hat_4 output; Wij input; Mii input; tsim input; u0 input; rho_hat_vec input
function d_beta_hat_4 = fcn(eps0, Wij, Mii, tsim, u0, rho_hat_vec)
%%%% 自适应律
iiuav = 4;
err_rho = Mii(iiuav, iiuav) * ( rho_hat_vec(:,iiuav) - u0(:) );
for jjuav = 1:5
    err_rho = err_rho + Wij(iiuav, jjuav) * ( rho_hat_vec(:,iiuav) - rho_hat_vec(:,jjuav) );
end
d_beta_hat_4 = ( err_rho(:)' ) * tanh( err_rho(:) ./ exp( -eps0 * tsim ) );

== matlab function sim_tnse_2024_pos_ctrl/update betai agent 5 ==
  data: eps0 input; d_beta_hat_5 output; Wij input; Mii input; tsim input; u0 input; rho_hat_vec input
function d_beta_hat_5 = fcn(eps0, Wij, Mii, tsim, u0, rho_hat_vec)
%%%% 自适应律
iiuav = 5;
err_rho = Mii(iiuav, iiuav) * ( rho_hat_vec(:,iiuav) - u0(:) );
for jjuav = 1:5
    err_rho = err_rho + Wij(iiuav, jjuav) * ( rho_hat_vec(:,iiuav) - rho_hat_vec(:,jjuav) );
end
d_beta_hat_5 = ( err_rho(:)' ) * tanh( err_rho(:) ./ exp( -eps0 * tsim ) );

== matlab function sim_tnse_2024_pos_ctrl/combine betai1 ==
  data: sigmai_1 input; sigmai_vec output; sigmai_2 input; sigmai_3 input; sigmai_4 input; sigmai_5 input
function sigmai_vec  = fcn(sigmai_1, sigmai_2, sigmai_3, sigmai_4, sigmai_5)
%%%% 合并分布式观测器变量
sigmai_vec = zeros(3,5);
sigmai_vec(:,1) = sigmai_1(:);
sigmai_vec(:,2) = sigmai_2(:);
sigmai_vec(:,3) = sigmai_3(:);
sigmai_vec(:,4) = sigmai_4(:);
sigmai_vec(:,5) = sigmai_5(:);

== matlab function sim_tnse_2024_pos_ctrl/update sigmai agent 1 ==
  data: kai0 input; lam0 input; eps0 input; d_sigmai_1 output; Wij input; Mii input; tsim input; u0 input; beta_hat_vec input; rho_hat_vec input; Phi_sec_sigma_vec input
function d_sigmai_1 = fcn(kai0, lam0, eps0, Wij, Mii, tsim, u0, beta_hat_vec, rho_hat_vec, Phi_sec_sigma_vec)
%%%% 求解分布式观测器变量
iiuav = 1;
err_rho = Mii(iiuav, iiuav) * ( rho_hat_vec(:,iiuav) - u0(:) );
for jjuav = 1:5
    err_rho = err_rho + Wij(iiuav, jjuav) * ( rho_hat_vec(:,iiuav) - rho_hat_vec(:,jjuav) );
end
d_sigmai_1 = -inv( Phi_sec_sigma_vec(:,:,iiuav) ) * ( ( kai0(:) ./ lam0(:) ) .* err_rho(:) ...
                                + ( beta_hat_vec(iiuav) ./ lam0(:) ) .* tanh( err_rho(:) ./ exp( -eps0 * tsim ) ) );

== matlab function sim_tnse_2024_pos_ctrl/update sigmai agent 2 ==
  data: kai0 input; lam0 input; eps0 input; d_sigmai_2 output; Wij input; Mii input; tsim input; u0 input; beta_hat_vec input; rho_hat_vec input; Phi_sec_sigma_vec input
function d_sigmai_2 = fcn(kai0, lam0, eps0, Wij, Mii, tsim, u0, beta_hat_vec, rho_hat_vec, Phi_sec_sigma_vec)
%%%% 求解分布式观测器变量
iiuav = 2;
err_rho = Mii(iiuav, iiuav) * ( rho_hat_vec(:,iiuav) - u0(:) );
for jjuav = 1:5
    err_rho = err_rho + Wij(iiuav, jjuav) * ( rho_hat_vec(:,iiuav) - rho_hat_vec(:,jjuav) );
end
d_sigmai_2 = -inv( Phi_sec_sigma_vec(:,:,iiuav) ) * ( ( kai0(:) ./ lam0(:) ) .* err_rho(:) ...
                                + ( beta_hat_vec(iiuav) ./ lam0(:) ) .* tanh( err_rho(:) ./ exp( -eps0 * tsim ) ) );

== matlab function sim_tnse_2024_pos_ctrl/update sigmai agent 3 ==
  data: kai0 input; lam0 input; eps0 input; d_sigmai_3 output; Wij input; Mii input; tsim input; u0 input; beta_hat_vec input; rho_hat_vec input; Phi_sec_sigma_vec input
function d_sigmai_3 = fcn(kai0, lam0, eps0, Wij, Mii, tsim, u0, beta_hat_vec, rho_hat_vec, Phi_sec_sigma_vec)
%%%% 求解分布式观测器变量
iiuav = 3;
err_rho = Mii(iiuav, iiuav) * ( rho_hat_vec(:,iiuav) - u0(:) );
for jjuav = 1:5
    err_rho = err_rho + Wij(iiuav, jjuav) * ( rho_hat_vec(:,iiuav) - rho_hat_vec(:,jjuav) );
end
d_sigmai_3 = -inv( Phi_sec_sigma_vec(:,:,iiuav) ) * ( ( kai0(:) ./ lam0(:) ) .* err_rho(:) ...
                                + ( beta_hat_vec(iiuav) ./ lam0(:) ) .* tanh( err_rho(:) ./ exp( -eps0 * tsim ) ) );

== matlab function sim_tnse_2024_pos_ctrl/update sigmai agent 4 ==
  data: kai0 input; lam0 input; eps0 input; d_sigmai_4 output; Wij input; Mii input; tsim input; u0 input; beta_hat_vec input; rho_hat_vec input; Phi_sec_sigma_vec input
function d_sigmai_4 = fcn(kai0, lam0, eps0, Wij, Mii, tsim, u0, beta_hat_vec, rho_hat_vec, Phi_sec_sigma_vec)
%%%% 求解分布式观测器变量
iiuav = 4;
err_rho = Mii(iiuav, iiuav) * ( rho_hat_vec(:,iiuav) - u0(:) );
for jjuav = 1:5
    err_rho = err_rho + Wij(iiuav, jjuav) * ( rho_hat_vec(:,iiuav) - rho_hat_vec(:,jjuav) );
end
d_sigmai_4 = -inv( Phi_sec_sigma_vec(:,:,iiuav) ) * ( ( kai0(:) ./ lam0(:) ) .* err_rho(:) ...
                                + ( beta_hat_vec(iiuav) ./ lam0(:) ) .* tanh( err_rho(:) ./ exp( -eps0 * tsim ) ) );

== matlab function sim_tnse_2024_pos_ctrl/update sigmai agent 5 ==
  data: kai0 input; lam0 input; eps0 input; d_sigmai_5 output; Wij input; Mii input; tsim input; u0 input; beta_hat_vec input; rho_hat_vec input; Phi_sec_sigma_vec input
function d_sigmai_5 = fcn(kai0, lam0, eps0, Wij, Mii, tsim, u0, beta_hat_vec, rho_hat_vec, Phi_sec_sigma_vec)
%%%% 求解分布式观测器变量
iiuav = 5;
err_rho = Mii(iiuav, iiuav) * ( rho_hat_vec(:,iiuav) - u0(:) );
for jjuav = 1:5
    err_rho = err_rho + Wij(iiuav, jjuav) * ( rho_hat_vec(:,iiuav) - rho_hat_vec(:,jjuav) );
end
d_sigmai_5 = -inv( Phi_sec_sigma_vec(:,:,iiuav) ) * ( ( kai0(:) ./ lam0(:) ) .* err_rho(:) ...
                                + ( beta_hat_vec(iiuav) ./ lam0(:) ) .* tanh( err_rho(:) ./ exp( -eps0 * tsim ) ) );

== matlab function sim_tnse_2024_pos_ctrl/cal rho_err_vec ==
  data: u0 input; rho_err_vec output; rho_hat_vec input
function rho_err_vec  = fcn(u0, rho_hat_vec)
%%%% 计算分布式观测误差
rho_err_vec = zeros(3,5);
for iiuav = 1:5
    rho_err_vec(:,iiuav) = u0(:) - rho_hat_vec(:,iiuav);
end

== matlab function sim_tnse_2024_pos_ctrl/update dpsy psy agent 2 ==
  data: Wij input; Mii input; d_2_psy_2 output; delta_ksi_vec input; delta_eta_vec input; ksi_i_vec input; eta_i_vec input; ksi_d_est_vec input; eta_d_est_vec input
function d_2_psy_2 = fcn(Wij, Mii, delta_ksi_vec, delta_eta_vec, ksi_i_vec, eta_i_vec, ksi_d_est_vec, eta_d_est_vec)
%%%% 计算集群构型估计二阶导数
iiuav = 2;
err_v_est = Mii(iiuav, iiuav) * ( eta_d_est_vec(:,iiuav) - ( eta_i_vec(:,iiuav) - delta_eta_vec(:,iiuav) ) );
err_p_est = Mii(iiuav, iiuav) * ( ksi_d_est_vec(:,iiuav) - ( ksi_i_vec(:,iiuav) - delta_ksi_vec(:,iiuav) ) );
for jjuav = 1:5
    err_v_est = err_v_est + Wij(iiuav, jjuav) * ( ( eta_d_est_vec(:,iiuav) - ( eta_i_vec(:,iiuav) - delta_eta_vec(:,iiuav) ) ) ...
                                                                                - ( eta_d_est_vec(:,jjuav) - ( eta_i_vec(:,jjuav) - delta_eta_vec(:,jjuav) ) ) );
    err_p_est = err_p_est + Wij(iiuav, jjuav) * ( ( ksi_d_est_vec(:,iiuav) - ( ksi_i_vec(:,iiuav) - delta_ksi_vec(:,iiuav) ) ) ...
                                                                                - ( ksi_d_est_vec(:,jjuav) - ( ksi_i_vec(:,jjuav) - delta_ksi_vec(:,jjuav) ) ) );
end
d_2_psy_2 = -err_v_est(:) - err_p_est(:);

== matlab function sim_tnse_2024_pos_ctrl/update dpsy psy agent 3 ==
  data: Wij input; Mii input; d_2_psy_3 output; delta_ksi_vec input; delta_eta_vec input; ksi_i_vec input; eta_i_vec input; ksi_d_est_vec input; eta_d_est_vec input
function d_2_psy_3 = fcn(Wij, Mii, delta_ksi_vec, delta_eta_vec, ksi_i_vec, eta_i_vec, ksi_d_est_vec, eta_d_est_vec)
%%%% 计算集群构型估计二阶导数
iiuav = 3;
err_v_est = Mii(iiuav, iiuav) * ( eta_d_est_vec(:,iiuav) - ( eta_i_vec(:,iiuav) - delta_eta_vec(:,iiuav) ) );
err_p_est = Mii(iiuav, iiuav) * ( ksi_d_est_vec(:,iiuav) - ( ksi_i_vec(:,iiuav) - delta_ksi_vec(:,iiuav) ) );
for jjuav = 1:5
    err_v_est = err_v_est + Wij(iiuav, jjuav) * ( ( eta_d_est_vec(:,iiuav) - ( eta_i_vec(:,iiuav) - delta_eta_vec(:,iiuav) ) ) ...
                                                                                - ( eta_d_est_vec(:,jjuav) - ( eta_i_vec(:,jjuav) - delta_eta_vec(:,jjuav) ) ) );
    err_p_est = err_p_est + Wij(iiuav, jjuav) * ( ( ksi_d_est_vec(:,iiuav) - ( ksi_i_vec(:,iiuav) - delta_ksi_vec(:,iiuav) ) ) ...
                                                                                - ( ksi_d_est_vec(:,jjuav) - ( ksi_i_vec(:,jjuav) - delta_ksi_vec(:,jjuav) ) ) );
end
d_2_psy_3 = -err_v_est(:) - err_p_est(:);

== matlab function sim_tnse_2024_pos_ctrl/update dpsy psy agent 4 ==
  data: Wij input; Mii input; d_2_psy_4 output; delta_ksi_vec input; delta_eta_vec input; ksi_i_vec input; eta_i_vec input; ksi_d_est_vec input; eta_d_est_vec input
function d_2_psy_4 = fcn(Wij, Mii, delta_ksi_vec, delta_eta_vec, ksi_i_vec, eta_i_vec, ksi_d_est_vec, eta_d_est_vec)
%%%% 计算集群构型估计二阶导数
iiuav = 4;
err_v_est = Mii(iiuav, iiuav) * ( eta_d_est_vec(:,iiuav) - ( eta_i_vec(:,iiuav) - delta_eta_vec(:,iiuav) ) );
err_p_est = Mii(iiuav, iiuav) * ( ksi_d_est_vec(:,iiuav) - ( ksi_i_vec(:,iiuav) - delta_ksi_vec(:,iiuav) ) );
for jjuav = 1:5
    err_v_est = err_v_est + Wij(iiuav, jjuav) * ( ( eta_d_est_vec(:,iiuav) - ( eta_i_vec(:,iiuav) - delta_eta_vec(:,iiuav) ) ) ...
                                                                                - ( eta_d_est_vec(:,jjuav) - ( eta_i_vec(:,jjuav) - delta_eta_vec(:,jjuav) ) ) );
    err_p_est = err_p_est + Wij(iiuav, jjuav) * ( ( ksi_d_est_vec(:,iiuav) - ( ksi_i_vec(:,iiuav) - delta_ksi_vec(:,iiuav) ) ) ...
                                                                                - ( ksi_d_est_vec(:,jjuav) - ( ksi_i_vec(:,jjuav) - delta_ksi_vec(:,jjuav) ) ) );
end
d_2_psy_4 = -err_v_est(:) - err_p_est(:);

== matlab function sim_tnse_2024_pos_ctrl/update dpsy psy agent 5 ==
  data: Wij input; Mii input; d_2_psy_5 output; delta_ksi_vec input; delta_eta_vec input; ksi_i_vec input; eta_i_vec input; ksi_d_est_vec input; eta_d_est_vec input
function d_2_psy_5 = fcn(Wij, Mii, delta_ksi_vec, delta_eta_vec, ksi_i_vec, eta_i_vec, ksi_d_est_vec, eta_d_est_vec)
%%%% 计算集群构型估计二阶导数
iiuav = 5;
err_v_est = Mii(iiuav, iiuav) * ( eta_d_est_vec(:,iiuav) - ( eta_i_vec(:,iiuav) - delta_eta_vec(:,iiuav) ) );
err_p_est = Mii(iiuav, iiuav) * ( ksi_d_est_vec(:,iiuav) - ( ksi_i_vec(:,iiuav) - delta_ksi_vec(:,iiuav) ) );
for jjuav = 1:5
    err_v_est = err_v_est + Wij(iiuav, jjuav) * ( ( eta_d_est_vec(:,iiuav) - ( eta_i_vec(:,iiuav) - delta_eta_vec(:,iiuav) ) ) ...
                                                                                - ( eta_d_est_vec(:,jjuav) - ( eta_i_vec(:,jjuav) - delta_eta_vec(:,jjuav) ) ) );
    err_p_est = err_p_est + Wij(iiuav, jjuav) * ( ( ksi_d_est_vec(:,iiuav) - ( ksi_i_vec(:,iiuav) - delta_ksi_vec(:,iiuav) ) ) ...
                                                                                - ( ksi_d_est_vec(:,jjuav) - ( ksi_i_vec(:,jjuav) - delta_ksi_vec(:,jjuav) ) ) );
end
d_2_psy_5 = -err_v_est(:) - err_p_est(:);

== matlab function sim_tnse_2024_pos_ctrl/choose rho_hat agent 1 ==
  data: x input; y output
function y = fcn(x)
iiuav = 1;
y = x(:,iiuav);

== matlab function sim_tnse_2024_pos_ctrl/cal ui agent 2 ==
  data: c1 input; c2 input; sat_sr_up input; sat_sr_low input; ui_2 output; rho_hat_vec input; dp_hat_vec input; si_vec input; ri_vec input
function ui_2 = fcn(c1, c2, sat_sr_up, sat_sr_low, rho_hat_vec, dp_hat_vec, si_vec, ri_vec)
%%%% 计算控制输入ui
iiuav = 2;
g0 = 9.80663;
e3 = [0;0;1];
sat_si_ri = zeros(3,1);
sat_ri = zeros(3,1);
c_mul_si_ri = c1 * ( si_vec(:,iiuav) + ri_vec(:,iiuav) );
c_mul_ri = c2 * ri_vec(:,iiuav);
for jj = 1:3
    if c_mul_si_ri(jj) < sat_sr_low(jj)
        sat_si_ri(jj) = sat_sr_low(jj);
    elseif c_mul_si_ri(jj) > sat_sr_up(jj)
        sat_si_ri(jj) = sat_sr_up(jj);
    else
        sat_si_ri(jj) = c_mul_ri(jj);
    end
    if c_mul_ri(jj) < sat_sr_low(jj)
        sat_ri(jj) = sat_sr_low(jj);
    elseif c_mul_ri(jj) > sat_sr_up(jj)
        sat_ri(jj) = sat_sr_up(jj);
    else
        sat_ri(jj) = c_mul_ri(jj);
    end
end
ui_2 = g0 * e3 + rho_hat_vec(:,iiuav) - dp_hat_vec(:,iiuav) ...
            - sat_si_ri(:) - sat_ri(:);

== matlab function sim_tnse_2024_pos_ctrl/cal ui agent 3 ==
  data: c1 input; c2 input; sat_sr_up input; sat_sr_low input; ui_3 output; rho_hat_vec input; dp_hat_vec input; si_vec input; ri_vec input
function ui_3 = fcn(c1, c2, sat_sr_up, sat_sr_low, rho_hat_vec, dp_hat_vec, si_vec, ri_vec)
%%%% 计算控制输入ui
iiuav = 3;
g0 = 9.80663;
e3 = [0;0;1];
sat_si_ri = zeros(3,1);
sat_ri = zeros(3,1);
c_mul_si_ri = c1 * ( si_vec(:,iiuav) + ri_vec(:,iiuav) );
c_mul_ri = c2 * ri_vec(:,iiuav);
for jj = 1:3
    if c_mul_si_ri(jj) < sat_sr_low(jj)
        sat_si_ri(jj) = sat_sr_low(jj);
    elseif c_mul_si_ri(jj) > sat_sr_up(jj)
        sat_si_ri(jj) = sat_sr_up(jj);
    else
        sat_si_ri(jj) = c_mul_ri(jj);
    end
    if c_mul_ri(jj) < sat_sr_low(jj)
        sat_ri(jj) = sat_sr_low(jj);
    elseif c_mul_ri(jj) > sat_sr_up(jj)
        sat_ri(jj) = sat_sr_up(jj);
    else
        sat_ri(jj) = c_mul_ri(jj);
    end
end
ui_3 = g0 * e3 + rho_hat_vec(:,iiuav) - dp_hat_vec(:,iiuav) ...
            - sat_si_ri(:) - sat_ri(:);

== matlab function sim_tnse_2024_pos_ctrl/cal ui agent 4 ==
  data: c1 input; c2 input; sat_sr_up input; sat_sr_low input; ui_4 output; rho_hat_vec input; dp_hat_vec input; si_vec input; ri_vec input
function ui_4 = fcn(c1, c2, sat_sr_up, sat_sr_low, rho_hat_vec, dp_hat_vec, si_vec, ri_vec)
%%%% 计算控制输入ui
iiuav = 4;
g0 = 9.80663;
e3 = [0;0;1];
sat_si_ri = zeros(3,1);
sat_ri = zeros(3,1);
c_mul_si_ri = c1 * ( si_vec(:,iiuav) + ri_vec(:,iiuav) );
c_mul_ri = c2 * ri_vec(:,iiuav);
for jj = 1:3
    if c_mul_si_ri(jj) < sat_sr_low(jj)
        sat_si_ri(jj) = sat_sr_low(jj);
    elseif c_mul_si_ri(jj) > sat_sr_up(jj)
        sat_si_ri(jj) = sat_sr_up(jj);
    else
        sat_si_ri(jj) = c_mul_ri(jj);
    end
    if c_mul_ri(jj) < sat_sr_low(jj)
        sat_ri(jj) = sat_sr_low(jj);
    elseif c_mul_ri(jj) > sat_sr_up(jj)
        sat_ri(jj) = sat_sr_up(jj);
    else
        sat_ri(jj) = c_mul_ri(jj);
    end
end
ui_4 = g0 * e3 + rho_hat_vec(:,iiuav) - dp_hat_vec(:,iiuav) ...
            - sat_si_ri(:) - sat_ri(:);

== matlab function sim_tnse_2024_pos_ctrl/cal ui agent 5 ==
  data: c1 input; c2 input; sat_sr_up input; sat_sr_low input; ui_5 output; rho_hat_vec input; dp_hat_vec input; si_vec input; ri_vec input
function ui_5 = fcn(c1, c2, sat_sr_up, sat_sr_low, rho_hat_vec, dp_hat_vec, si_vec, ri_vec)
%%%% 计算控制输入ui
iiuav = 5;
g0 = 9.80663;
e3 = [0;0;1];
sat_si_ri = zeros(3,1);
sat_ri = zeros(3,1);
c_mul_si_ri = c1 * ( si_vec(:,iiuav) + ri_vec(:,iiuav) );
c_mul_ri = c2 * ri_vec(:,iiuav);
for jj = 1:3
    if c_mul_si_ri(jj) < sat_sr_low(jj)
        sat_si_ri(jj) = sat_sr_low(jj);
    elseif c_mul_si_ri(jj) > sat_sr_up(jj)
        sat_si_ri(jj) = sat_sr_up(jj);
    else
        sat_si_ri(jj) = c_mul_ri(jj);
    end
    if c_mul_ri(jj) < sat_sr_low(jj)
        sat_ri(jj) = sat_sr_low(jj);
    elseif c_mul_ri(jj) > sat_sr_up(jj)
        sat_ri(jj) = sat_sr_up(jj);
    else
        sat_ri(jj) = c_mul_ri(jj);
    end
end
ui_5 = g0 * e3 + rho_hat_vec(:,iiuav) - dp_hat_vec(:,iiuav) ...
            - sat_si_ri(:) - sat_ri(:);

== matlab function sim_tnse_2024_pos_ctrl/cal si agent 2 ==
  data: Wij input; Mii input; si_2 output; delta_ksi_vec input; ksi0 input; ksi_i_vec input; ksi_d_est_vec input
function si_2 = fcn(Wij, Mii, delta_ksi_vec, ksi0, ksi_i_vec, ksi_d_est_vec)
%%%% 计算位置误差面
iiuav = 2;
si_2 = Mii(iiuav, iiuav) * ( ksi_i_vec(:,iiuav) - ksi0(:) - delta_ksi_vec(:,iiuav) ) ...
            + Mii(iiuav, iiuav) * ( ksi_d_est_vec(:,iiuav) - ksi0(:) );
for jjuav = 1:5
    si_2 = si_2 + Wij(iiuav, jjuav) * ( ( ksi_i_vec(:,iiuav) - delta_ksi_vec(:,iiuav) ) - ( ksi_i_vec(:,jjuav) - delta_ksi_vec(:,jjuav) ) ) ...
                        + Wij(iiuav, jjuav) * ( ksi_d_est_vec(:,iiuav) - ksi_d_est_vec(:,jjuav) );
end

== matlab function sim_tnse_2024_pos_ctrl/combine formation control input ==
  data: eta_i_vec output; ksi_i_vec output; eta_1 input; eta_2 input; eta_3 input; eta_4 input; eta_5 input; ksi_1 input; ksi_2 input; ksi_3 input; ksi_4 input; ksi_5 input
function [eta_i_vec, ksi_i_vec] = fcn(eta_1, eta_2, eta_3, eta_4, eta_5, ...
                                                                ksi_1, ksi_2, ksi_3, ksi_4, ksi_5)
%%%% 合并领导者编队跟踪误差结果
eta_i_vec = [eta_1(:), eta_2(:), eta_3(:), eta_4(:), eta_5(:)];
ksi_i_vec = [ksi_1(:), ksi_2(:), ksi_3(:), ksi_4(:), ksi_5(:)];

== matlab function sim_tnse_2024_pos_ctrl/choose rho_hat agent 2 ==
  data: x input; y output
function y = fcn(x)
iiuav = 2;
y = x(:,iiuav);

== matlab function sim_tnse_2024_pos_ctrl/choose rho_hat agent 3 ==
  data: x input; y output
function y = fcn(x)
iiuav = 3;
y = x(:,iiuav);

== matlab function sim_tnse_2024_pos_ctrl/choose rho_hat agent 4 ==
  data: x input; y output
function y = fcn(x)
iiuav = 4;
y = x(:,iiuav);

== matlab function sim_tnse_2024_pos_ctrl/choose rho_hat agent 5 ==
  data: x input; y output
function y = fcn(x)
iiuav = 5;
y = x(:,iiuav);

== matlab function sim_tnse_2024_pos_ctrl/uav translational dynamics agent 1 ==
  data: dvi output; Ri input; ui_vec input; dpi_vec input
function dvi = fcn(Ri, ui_vec, dpi_vec)
%%%% 根据有限时间控制输入计算无人机平移动力学微分方程
iiuav = 1;
g0 = 9.80663;
e3 = [0;0;1];
ui = ui_vec(:,iiuav);
dvi = -g0 * e3 + norm(ui,2) * Ri(:,:,iiuav) * e3 + dpi_vec(:,iiuav);

== matlab function sim_tnse_2024_pos_ctrl/uav translational dynamics agent 2 ==
  data: dvi output; Ri input; ui_vec input; dpi_vec input
function dvi = fcn(Ri, ui_vec, dpi_vec)
%%%% 根据有限时间控制输入计算无人机平移动力学微分方程
iiuav = 2;
g0 = 9.80663;
e3 = [0;0;1];
ui = ui_vec(:,iiuav);
dvi = -g0 * e3 + norm(ui,2) * Ri(:,:,iiuav) * e3 + dpi_vec(:,iiuav);

== matlab function sim_tnse_2024_pos_ctrl/uav translational dynamics agent 3 ==
  data: dvi output; Ri input; ui_vec input; dpi_vec input
function dvi = fcn(Ri, ui_vec, dpi_vec)
%%%% 根据有限时间控制输入计算无人机平移动力学微分方程
iiuav = 3;
g0 = 9.80663;
e3 = [0;0;1];
ui = ui_vec(:,iiuav);
dvi = -g0 * e3 + norm(ui,2) * Ri(:,:,iiuav) * e3 + dpi_vec(:,iiuav);

== matlab function sim_tnse_2024_pos_ctrl/uav translational dynamics agent 4 ==
  data: dvi output; Ri input; ui_vec input; dpi_vec input
function dvi = fcn(Ri, ui_vec, dpi_vec)
%%%% 根据有限时间控制输入计算无人机平移动力学微分方程
iiuav = 4;
g0 = 9.80663;
e3 = [0;0;1];
ui = ui_vec(:,iiuav);
dvi = -g0 * e3 + norm(ui,2) * Ri(:,:,iiuav) * e3 + dpi_vec(:,iiuav);

== matlab function sim_tnse_2024_pos_ctrl/uav translational dynamics agent 5 ==
  data: dvi output; Ri input; ui_vec input; dpi_vec input
function dvi = fcn(Ri, ui_vec, dpi_vec)
%%%% 根据有限时间控制输入计算无人机平移动力学微分方程
iiuav = 5;
g0 = 9.80663;
e3 = [0;0;1];
ui = ui_vec(:,iiuav);
dvi = -g0 * e3 + norm(ui,2) * Ri(:,:,iiuav) * e3 + dpi_vec(:,iiuav);

== matlab function sim_tnse_2024_pos_ctrl/cal Ri ==
  data: Ri output; Rei input; Rci input
function Ri = fcn(Rei, Rci)
%%%% 使用罗德里格公式由四元数Qci求解Rci
Ri = zeros(3,3,5);
for iiuav = 1:5
    Ri(:,:,iiuav) = Rci(:,:,iiuav) * Rei(:,:,iiuav);
end

end
